simulink model "robot_LAB__2"  (R2024b)
settings: Solver=FixedStepAuto  StartTime=0.0  StopTime=total_time  RelTol=1e-3
values from neighbouring files (symbols this model uses):
  D = diag([0.001, 0.001, 0.0175/6, 0.0175/6, 0.0175/6, 0.0175/6*Ts, 0.0175/6*Ts].^2)    [init_LAB__2.m]
  d = 0.165    [init_LAB__3.m]
  d_nom = 0.165    [MAIN_ROBOT.m]    (also in init_LAB__2.m)
  mode = 2    [MAIN_ROBOT.m]    (also in init_LAB__2.m)
  omega_max = 10    [MAIN_ROBOT.m]    (also in init_LAB__2.m)
  omega_trj = 2*pi    (= 6.28318530718)    [MAIN_ROBOT.m]    (also in init_LAB__2.m)
  P_INIT_EKF = diag([0.001, 0.001, 0.0175/6, 0.0175/6, 0.0175/6, 0.0175/6*Ts, 0.0175/6*Ts].^2)    [init_LAB__2.m]
  prob_gps_loss = 0.99    [init_LAB__2.m]
  r = 0.03    [init_LAB__3.m]
  R = 0.4    [MAIN_ROBOT.m]    (also in init_LAB__2.m)
  R_2 = diag([ENCODER_QUANTIZATION/6,ENCODER_QUANTIZATION/6].^2)    [init_LAB__2.m]
  R_3 = diag(([0.001, ENCODER_QUANTIZATION/6,ENCODER_QUANTIZATION/6]).^2)    [init_LAB__2.m]
  R_4 = diag(([0.001, 0.001, ENCODER_QUANTIZATION/6,ENCODER_QUANTIZATION/6]).^2)    [init_LAB__2.m]
  R_5 = diag(([0.001, 0.001, 0.001, ENCODER_QUANTIZATION/6,ENCODER_QUANTIZATION/6]).^2)    [init_LAB__2.m]
  r_nom = 0.03    [MAIN_ROBOT.m]    (also in init_LAB__2.m)
  T_s = 0.04    [id_template.m]    (also in id_template_ED.m)
  Ta = 1    [MAIN_ROBOT.m]    (also in init_LAB__2.m)
  Tc = 30    [MAIN_ROBOT.m]    (also in init_LAB__2.m = 45)
  total_time = 40    [MAIN_ROBOT.m]    (also in init_LAB__2.m = 47)
  Ts = 0.04    [MAIN_ROBOT.m]    (also in init_LAB__2.m)
  Z_INIT_EKF = [1; 1; 0; 0; 0; 0; 0]    [init_LAB__2.m]
undefined symbols (not defined in the file or in its folder): X, Y
libraries: robotlib x4
settings Model: Creator=leontecosm  LastModifiedBy=leontecosm
settings OptimizationCC: DefaultParameterBehavior=Inlined  EnhancedBackFolding=on  PassReuseOutputArgsAs=Individual arguments  ZeroExternalMemoryAtStartup=off  ZeroInternalMemoryAtStartup=off  MaxStackSize=64  OptimizeBlockOrder=speed  DifferentSizesBufferReuse=on  OptimizationCustomize=off  EfficientTunableParamExpr=on
settings DebuggingCC: ParameterTunabilityLossMsg=error
settings HardwareCC: ProdBitPerPointer=32  ProdBitPerSizeT=32  ProdBitPerPtrDiffT=32  ProdLargestAtomicFloat=None  ProdIntDivRoundTo=Undefined  ProdEndianess=Unspecified  ProdWordSize=32  ProdHWDeviceType=Generic->Unspecified (assume 32-bit Generic)
settings SFSimCC: MATLABDynamicMemAlloc=off
settings RTWCC: Description=Embedded Coder  SystemTargetFile=ert.tlc  HardwareBoard=Robot Operating System (ROS)  TLCOptions="-aInlineSetEventsForThisBaseRateFcn=TLC_FALSE -aSuppressMultiTaskScheduler=TLC_FALSE  -aRateBasedStepFcn=0"  TemplateMakefile=ert_default_tmf  Toolchain=Catkin  TargetLang=C++
settings CodeAppCC: ForceParamTrailComments=on  IgnoreCustomStorageClasses=off  OperatorAnnotations=on  SimulinkDataObjDesc=on  SFDataObjDesc=on  InsertBlockDesc=on

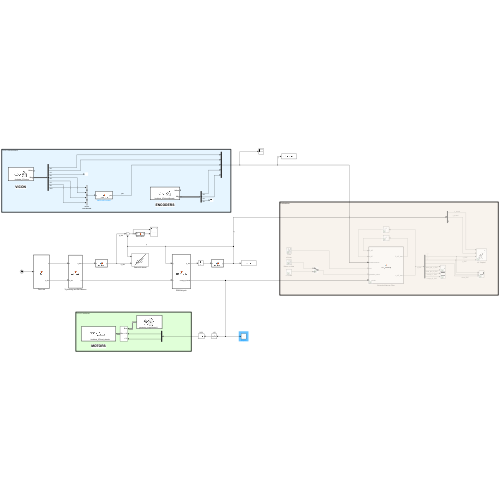
[thumbnail: Simulink's stored preview of the top-level diagram]
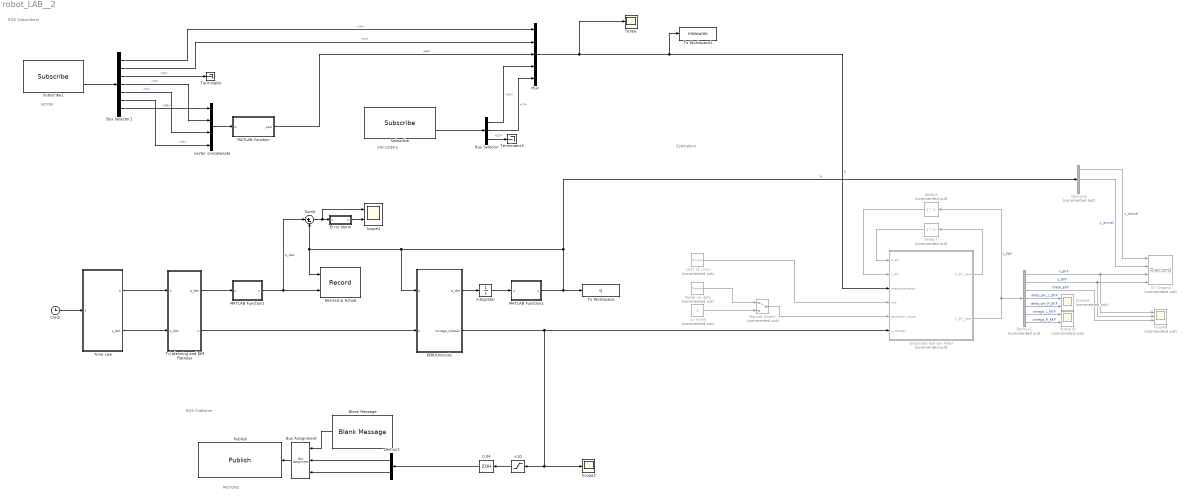
== system robot_LAB__2 ==
  note: Estimation
  note: ENCODERS
  note: ROS Publisher
  note: ROS Subscribers
  note: VICON
  note: MOTORS
  " Loss of vicon" : UniformRandomNumber  Commented=on  Minimum=0
  0.04 : ZeroOrderHold  SampleTime=Ts
  <10 : Saturate  UpperLimit=omega_max  LowerLimit=-omega_max
  Blank Message : robotlib/Blank Message  messageClass=Message  entityType=geometry_msgs/Vector3  messageType=geometry_msgs/Vector3  SampleTime=Ts  legacyBusStruct=off
      settings: LibrarySourceBlock=roslib/ROS/Blank Message
  Bus Assignment : BusAssignment  AssignedSignals=X,Y
  Bus Selector : BusSelector  OutputSignals=X,Y,Z
  Bus Selector1 : BusSelector  OutputSignals=Pose.Pose.Position.X,Pose.Pose.Position.Y,Pose.Pose.Position.Z,Pose.Pose.Orientation.X,Pose.Pose.Orientation.Y,Pose.Pose.Orientation.Z,Pose.Pose.Orientation.W
  Clock : Clock
      settings: Decimation=1/Ts
  DDR/Unicycle : MATLAB Function  TreatAsAtomicUnit=on
  Delay6 : Delay  Commented=on  DelayLength=1  InitialCondition=Z_INIT_EKF
  Delay7 : Delay  Commented=on  DelayLength=1  InitialCondition=P_INIT_EKF
  Demux1 : Demux  Commented=on  Outputs=7
  Demux2 : Demux  Outputs=2
  Demux6 : Demux  Commented=on  Outputs=3
  Desired & Actual : Record  FileSettingsInternal="{\"entries\":[{\"content\":{\"excelSettings\":{\"content\":{},\"type\":\"Streamout.ExcelSettings\"}},\"type\":\"Streamout.FileSettingStorage\",\"uuid\":\"\"}],\"packageUris\":[\"http:\\/\\/schema.mathworks.com\\/mf0\\/streamout_blocks\\/R2020a\"],\"version\":\"1.0\"}"  Layout=[2 1]  SignalsInternal="{\"entries\":[{\"content\":{\"signals\":[{\"content\":{\"blockPath\":[],\"dimensions\":[1,3],\"domain\":\"\",\"hasChildren\":true,\"lineColor\":\"#77ac30\",\"lineWidth\":2,\"port\":1,\"sid\":[\"\"],\"signalID\":1,\"signalName\":\"q\"},\"type\":\"RecordBlkView.Signal\",\"uuid\":\"\"},{\"content\":{\"blockPath\":[],\"channel\":[1,1],\"dimensions\":[1,3],\"domain\":\"\",\"lineColor\":\"#139fff\",\"lineWidth\":2,\"parentID\":1,\"port\":1,\"sid\":[\"\"],\"signalID\":2,\"signalName\":\"q\"},\"type\":\"RecordBlkView.Signal\",\"uuid\":\"\"},{\"content\":{\"blockPath\":[],\"dimensions\":[1,3],\"domain\":\"\",\"hasChildren\":true,\"lineColor\":\"#a2142f\",\"lineWidth\":2,\"port\":2,\"sid\":[\"\"],\"signalID\":3,\"signalName\":\"q_des\"},\"type\":\"RecordBlkView.Signal\",\"uuid\":\"\"},{\"content\":{\"blockPath\":[],\"channel\":[1,1],\"dimensions\":[1,3],\"domain\":\"\",\"lineColor\":\"#b746ff\",\"lineWidth\":2,\"parentID\":3,\"plots\":[ 1 ],\"port\":2,\"sid\":[\"\"],\"signalID\":4,\"signalName\":\"q_des\"},\"type\":\"RecordBlkView.Signal\",\"uuid\":\"\"},{\"content\":{\"blockPath\":[],\"channel\":[1,2],\"dimensions\":[1,3],\"domain\":\"\",\"lineColor\":\"#a2142f\",\"lineWidth\":2,\"parentID\":1,\"port\":1,\"sid\":[\"\"],\"signalID\":5,\"signalName\":\"q\"},\"type\":\"RecordBlkView.Signal\",\"uuid\":\"\"},{\"content\":{\"blockPath\":[],\"channel\":[1,3],\"dimensions\":[1,3],\"domain\":\"\",\"lineColor\":\"#139fff\",\"lineWidth\":2,\"parentID\":1,\"port\":1,\"sid\":[\"\"],\"signalID\":6,\"signalName\":\"q\"},\"type\":\"RecordBlkView.Signal\",\"uuid\":\"\"},{\"content\":{\"blockPath\":[],\"channel\":[1,2],\"dimensions\":[1,3],\"domain\":\"\",\"lineColor\":\"#ff6929\",\"lineWidth\":2,\"parentID\":3,\"plots\":[ 1 ],\"port\":2,\"sid\":[\"\"],\"signalID\":7,\"signalName\":\"q_des\"},\"type\":\"RecordBlkView.Signal\",\"uuid\":\"\"},{\"content\":{\"blockPath\":[],\"channel\":[1,3],\"dimensions\":[1,3],\"domain\":\"\",\"lineColor\":\"#b746ff\",\"lineWidth\":2,\"parentID\":3,\"plots\":[ 2 ],\"port\":2,\"sid\":[\"\"],\"signalID\":8,\"signalName\":\"q_des\"},\"type\":\"RecordBlkView.Signal\",\"uuid\":\"\"}]},\"type\":\"RecordBlkView.InputSignals\",\"uuid\":\"\"}],\"packageUris\":[\"http:\\/\\/schema.mathworks.com\\/mf0\\/streamout_blocks\\/R2020a\"],\"version\":\"1.0\"}"  VisualizationBindings="{\"xyplotplugin\":{\"info\":[{\"series\":[{\"bindingParametersList\":[{\"parameter\":\"X-Axis\",\"signalID\":4,\"signalName\":\"q_des(1,1)\"},{\"parameter\":\"Y-Axis\",\"signalID\":7,\"signalName\":\"q_des(1,2)\"}],\"seriesID\":0}],\"subplotID\":1}]}}"  CompatibilityTag=XY
  Error Norm : MATLAB Function  TreatAsAtomicUnit=on
  Extended Kalman Filter : MATLAB Function  Commented=on  TreatAsAtomicUnit=on
  Integrator : Integrator  InitialCondition=[0;0;atan(1/2)]
  MATLAB Function : MATLAB Function  TreatAsAtomicUnit=on
  MATLAB Function1 : MATLAB Function  TreatAsAtomicUnit=on
  MATLAB Function2 : MATLAB Function  TreatAsAtomicUnit=on
  Manual Switch : ManualSwitch  Commented=on
  Mux : Mux  Inputs=5
  Noise on data : RandomNumber  Commented=on  Variance=0.0001
  Publish : robotlib/Publish  topicSource=Specify your own  topic=/turtlebot_07/cmd_wheels  messageType=geometry_msgs/Vector3  legacyBusStruct=off  messageQueueLength=1
      settings: LibrarySourceBlock=roslib/ROS/Publish
  Scope : Scope
  Scope1 : Scope  NumInputPorts=2
  Scope10 : Scope  Commented=on  NumInputPorts=2
  Scope2 : Scope
  Scope8 : Scope  Commented=on  NumInputPorts=3
  Scope9 : Scope  Commented=on  NumInputPorts=2
  Subscribe : robotlib/Subscribe  topicSource=Specify your own  topic=/turtlebot_07/wheelSpeeds  messageType=geometry_msgs/Vector3  SampleTime=-1  legacyBusStruct=off  messageQueueLength=1
      settings: LibrarySourceBlock=roslib/ROS/Subscribe
  Subscribe1 : robotlib/Subscribe  topicSource=Specify your own  topic=/turtlebot_07/odom  messageType=nav_msgs/Odometry  SampleTime=-1  legacyBusStruct=off  messageQueueLength=1
      settings: LibrarySourceBlock=roslib/ROS/Subscribe
  Sum5 : Sum  Inputs=|+-
  Terminator : Terminator
  Terminator3 : Terminator
  Time Law : MATLAB Function  TreatAsAtomicUnit=on
  To Workspace : ToWorkspace  VariableName=q  SaveFormat=Structure With Time  SampleTime=-1
  To Workspace1 : ToWorkspace  VariableName=measures  SaveFormat=Structure With Time  SampleTime=-1
  Trj planning and Diff Flatness : MATLAB Function  TreatAsAtomicUnit=on
  XY Graph4 : Record  Commented=on  FileSettingsInternal="{\"entries\":[{\"content\":{\"excelSettings\":{\"content\":{},\"type\":\"Streamout.ExcelSettings\"}},\"type\":\"Streamout.FileSettingStorage\",\"uuid\":\"\"}],\"packageUris\":[\"http:\\/\\/schema.mathworks.com\\/mf0\\/streamout_blocks\\/R2020a\"],\"version\":\"1.0\"}"  Layout=[1 1]  SignalsInternal="{\"entries\":[{\"content\":{\"signals\":[{\"content\":{\"blockPath\":[],\"dimensions\":[1,1],\"domain\":\"\",\"lineColor\":\"#0072bd\",\"lineWidth\":2,\"plots\":[ 1 ],\"port\":1,\"signalID\":1,\"signalName\":\"x_actual\"},\"type\":\"RecordBlkView.Signal\",\"uuid\":\"\"},{\"content\":{\"blockPath\":[],\"dimensions\":[1,1],\"domain\":\"\",\"lineColor\":\"#d95319\",\"lineWidth\":2,\"plots\":[ 1 ],\"port\":2,\"signalID\":2,\"signalName\":\"y_actual\"},\"type\":\"RecordBlkView.Signal\",\"uuid\":\"\"},{\"content\":{\"blockPath\":[],\"dimensions\":[1,1],\"domain\":\"\",\"lineColor\":\"#edb120\",\"lineWidth\":2,\"plots\":[ 1 ],\"port\":3,\"signalID\":3,\"signalName\":\"x_EKF\"},\"type\":\"RecordBlkView.Signal\",\"uuid\":\"\"},{\"content\":{\"blockPath\":[],\"dimensions\":[1,1],\"domain\":\"\",\"lineColor\":\"#7e2f8e\",\"lineWidth\":2,\"plots\":[ 1 ],\"port\":4,\"signalID\":4,\"signalName\":\"y_EKF\"},\"type\":\"RecordBlkView.Signal\",\"uuid\":\"\"}]},\"type\":\"RecordBlkView.InputSignals\",\"uuid\":\"\"}],\"packageUris\":[\"http:\\/\\/schema.mathworks.com\\/mf0\\/streamout_blocks\\/R2020a\"],\"version\":\"1.0\"}"  VisualizationBindings="{\"xyplotplugin\":{\"info\":[{\"series\":[{\"bindingParametersList\":[{\"parameter\":\"X-Axis\",\"signalID\":1,\"signalName\":\"x_actual\"},{\"parameter\":\"Y-Axis\",\"signalID\":2,\"signalName\":\"y_actual\"}],\"seriesID\":0},{\"bindingParametersList\":[{\"parameter\":\"X-Axis\",\"signalID\":3,\"signalName\":\"x_EKF\"},{\"parameter\":\"Y-Axis\",\"signalID\":4,\"signalName\":\"y_EKF\"}],\"seriesID\":1}],\"subplotID\":1}]}}"  CompatibilityTag=XY
  no noise : Constant  Commented=on
  vector concatenate : Concatenate  NumInputs=4
  wires:
  Integrator/1 -> MATLAB Function2/1(u)
  Sum5/1 -> Scope1/1, Error Norm/1(u)
  DDR/Unicycle/1(q_dot) -> Integrator/1
  Trj planning and Diff Flatness/2(u) -> DDR/Unicycle/2(u)
  Demux2/1 -> Bus Assignment/2
  Time Law/1(s) -> Trj planning and Diff Flatness/1(s)
  Time Law/2(s_dot) -> Trj planning and Diff Flatness/2(s_dot)
  Clock/1 -> Time Law/1(t)
  Error Norm/1(y) -> Scope1/2
  <10/1 -> 0.04/1
  Blank Message/1 -> Bus Assignment/1
  Bus Assignment/1 -> Publish/1
  Demux2/2 -> Bus Assignment/3
  Subscribe/2 -> Bus Selector/1
  MATLAB Function/1(yaw) -> Mux/3  "yaw"
  Bus Selector1/4 -> vector concatenate/2  "<X>"
  Bus Selector/1 -> Mux/4  "<X>"
  Bus Selector1/5 -> vector concatenate/3  "<Y>"
  Bus Selector1/1 -> Mux/1  "<X>"
  Bus Selector1/6 -> vector concatenate/4  "<Z>"
  Bus Selector/2 -> Mux/5  "<Y>"
  Bus Selector1/2 -> Mux/2  "<Y>"
  Subscribe1/2 -> Bus Selector1/1
  vector concatenate/1 -> MATLAB Function/1(q)
  Bus Selector1/7 -> vector concatenate/1  "<W>"
  Bus Selector1/3 -> Terminator/1  "<Z>"
  Bus Selector/3 -> Terminator3/1  "<Z>"
  Trj planning and Diff Flatness/1(q_des) -> MATLAB Function1/1(u)
  MATLAB Function1/1(y) -> Desired & Actual/2, Sum5/1  "q_des"
  0.04/1 -> Demux2/1
  Demux1/3 -> Scope8/3  "theta_EKF"
  Demux1/6 -> Scope10/1  "omega_L_EKF"
  Delay7/1 -> Extended Kalman Filter/1(P_KF)
  Demux1/2 -> Scope8/2, XY Graph4/4  "y_EKF"
  Extended Kalman Filter/2(z_KF_new) -> Demux1/1, Delay6/1  "z_EKF"
  Demux6/2 -> XY Graph4/2  "y_actual"
  Demux6/1 -> XY Graph4/1  "x_actual"
  MATLAB Function2/1(y) -> Demux6/1, DDR/Unicycle/1(q), Desired & Actual/1, Sum5/2, To Workspace/1  "q"
  Extended Kalman Filter/1(P_KF_new) -> Delay7/1
  Demux1/4 -> Scope9/1  "delta_phi_L_EKF"
  Demux1/1 -> Scope8/1, XY Graph4/3  "x_EKF"
  DDR/Unicycle/2(omega_wheels) -> Extended Kalman Filter/6(u_wheels), <10/1, Scope2/1
  Demux1/7 -> Scope10/2  "omega_R_EKF"
  Noise on data/1 -> Manual Switch/1
  Delay6/1 -> Extended Kalman Filter/2(z_KF)
  Demux1/5 -> Scope9/2  "delta_phi_R_EKF"
  Manual Switch/1 -> Extended Kalman Filter/5(gaussian_noise)
  no noise/1 -> Manual Switch/2
  " Loss of vicon"/1 -> Extended Kalman Filter/4(rnd)
  Mux/1 -> Scope/1, Extended Kalman Filter/3(messurements), To Workspace1/1  "q"

== matlab function robot_LAB__2/MATLAB Function ==
  data: q input; yaw output
function yaw = quat2yaw(q)

% normalize to avoid issues
q = q / norm(q);

w = q(1);
x = q(2);
y = q(3);
z = q(4);

% rotation around Z axis
yaw = atan2(2*(w*z + x*y), 1 - 2*(y^2 + z^2));

end

== matlab function robot_LAB__2/Time Law ==
  data: t input; s output; s_dot output; total_time parameter; mode parameter; Ta parameter; Tc parameter
function [s, s_dot] = fcn(t,total_time, mode,Ta, Tc)
s=0;
s_dot=0;

if mode==1%if mode =1 costasnt time law else trapezoidal
    s_dot = 1/total_time;
    s=t/total_time;
else
   

    Vc=1/(Ta+Tc);% velocità costante
    a=Vc/Ta;% acceleration
    
    switch 1 %formula on the slide
        case t<Ta
            s_dot=a*t;
            s=(a*(t^2))/2;

        case (t>=Ta)&&(t<(Tc+Ta))
            s_dot=Vc;
            s=(a*(Ta^2))/2+Vc*(t-Ta);

        case (t>=(Tc+Ta))&&(t<(Tc+2*Ta))
            s_dot=Vc-a*(t-Ta-Tc);
            s=(a*(Ta^2))/2+Vc*Tc+Vc*(t-Ta-Tc)-a*(t-Ta-Tc)^2/2;

        case t>=(Tc+2*Ta)
            s_dot=0;
            s=1;
    end

end

== matlab function robot_LAB__2/DDR//Unicycle ==
  data: q input; u input; q_dot output; omega_wheels output; d_nom parameter; r_nom parameter
function [q_dot, omega_wheels] = DDR_Unicycle(q, u, d_nom, r_nom)
v = u(1);
omega = u(2);
q_dot = [cos(q(3))*v; sin(q(3))*v; omega];

%evaluation of speed wheels
omega_L = (2*v - d_nom*omega) / (2*r_nom);
omega_R = (2*v + d_nom*omega) / (2*r_nom);
omega_wheels=[omega_R; omega_L];

== matlab function robot_LAB__2/Trj planning and Diff Flatness ==
  data: q_des output; u output; R parameter; omega_trj parameter; s input; s_dot input
function [q_des, u] = get_inputs(R,omega_trj, s, s_dot)

x=R*sin(2*omega_trj.*s);
y=R*sin(omega_trj.*s);

x_dot = R*2*omega_trj*cos(2*omega_trj.*s);
y_dot = R*omega_trj*cos(omega_trj.*s);

x_ddot = R*4*omega_trj*omega_trj*(-sin(2*omega_trj.*s));
y_ddot = R*omega_trj*omega_trj*(-sin(omega_trj.*s));

theta = atan2(y_dot,x_dot);

%   v
v = s_dot*sqrt(y_dot^2 + x_dot^2);

%   omega
w = s_dot*(x_dot*y_ddot - y_dot*x_ddot)/(y_dot^2 + x_dot^2);
    
q_des = [x; y; theta];

u = [v; w];

== matlab function robot_LAB__2/Error Norm ==
  data: u input; y output
function y = e_norm(u)

y = sqrt(sum(u(1:2).^2));

== matlab function robot_LAB__2/MATLAB Function2 ==
  data: u input; y output
function y = wrapToPi(u)
theta = wrapToPi(u(3));
y = [u(1),u(2),theta];

== matlab function robot_LAB__2/MATLAB Function1 ==
  data: u input; y output
function y = wrapToPi(u)
theta = wrapToPi(u(3));
y = [u(1),u(2),theta];

== matlab function robot_LAB__2/Extended Kalman Filter ==
  data: P_KF input; P_KF_new output; z_KF input; messurements input; D parameter; R_2 parameter; R_3 parameter; R_4 parameter; R_5 parameter; T_s parameter; r parameter; d parameter; prob_gps_loss parameter; rnd input; gaussian_noise input; z_KF_new output; u_wheels input
function [P_KF_new, z_KF_new] = EKF_filtering(P_KF, z_KF, messurements, D, R_2, R_3, R_4, R_5 ,T_s, r, d, prob_gps_loss, rnd, gaussian_noise,u_wheels)

% z_KF = [x_EKF, y_EKF, theta_EKF, delta_phi_L_EKF, delta_phi_R_EKF, omega_L_EKF, omega_R_EKF]

v_k = r * (z_KF(6) + z_KF(7))/2;
w_k = r * (z_KF(7) - z_KF(6))/d;

theta_mean = z_KF(3) + (w_k * T_s)/2;

F_k = [1, 0, -T_s * v_k * sin(theta_mean), 0, 0, T_s * r * cos(theta_mean)/2 + (T_s)^2 * r * v_k * sin(theta_mean)/(2*d), T_s * r * cos(theta_mean)/2 - (T_s)^2 * r * v_k * sin(theta_mean)/(2*d);
    0, 1, T_s * v_k * cos(theta_mean), 0, 0, T_s * r * sin(theta_mean)/2 - (T_s)^2 * r * v_k * cos(theta_mean)/(2*d), T_s * r * sin(theta_mean)/2 + (T_s)^2 * r * v_k * cos(theta_mean)/(2*d);
    0, 0, 1, 0, 0, (-T_s*r)/d, (T_s*r)/d;
    0, 0, 0, 0, 0, T_s, 0;
    0, 0, 0, 0, 0, 0, T_s;
    0, 0, 0, 0, 0, 0, 0;
    0, 0, 0, 0, 0, 0, 0];

%% Prediction part

z_pred = [z_KF(1)+(T_s*r*(z_KF(6)+z_KF(7))/2)*cos(theta_mean + (T_s*r*(z_KF(6)+z_KF(7)))/(2*d));
    z_KF(2)+(T_s*r*(z_KF(6)+z_KF(7))/2)*sin(theta_mean + (T_s*r*(z_KF(7)-z_KF(6)))/(2*d));
    theta_mean + (T_s*r*(z_KF(7)-z_KF(6))/(2*d));
    T_s*z_KF(6);
    T_s*z_KF(7);
    u_wheels(1);
    u_wheels(2)];

P_pred = F_k * P_KF * F_k' + D;


%% Update

if(rnd<prob_gps_loss) 

    % Just encoders
    y_messurement = [messurements(1); messurements(2)];
    H = [0, 0, 0, 1, 0, 0, 0;
        0, 0, 0, 0, 1, 0, 0];

    e = y_messurement - H * z_pred;
    K = P_pred * H' /(H * P_pred * H' + R_2);

    z_KF_new = z_pred +  K * e;
    P_KF_new = P_pred - K * H * P_pred;

else 
    % GPS(x,y,yaw) + Encoders(omegaL,omegaR)
    y_messurement = [messurements(3)+gaussian_noise;messurements(4)+gaussian_noise; messurements(1); messurements(2)];

    H = [1, 0, 0, 0, 0, 0, 0;
         0, 1, 0, 0, 0, 0, 0;
         0, 0, 1, 0, 0, 0, 0;
         0, 0, 0, 0, 0, 1, 0;
         0, 0, 0, 0, 0, 0, 1];

    e = y_messurement - H * z_pred;
    K = P_pred * H' /(H * P_pred * H' + R_5);

    z_KF_new = z_pred + K * e;
    P_KF_new = P_pred - K * H * P_pred;

end
